simulink model "simu_pi"  (R2020b)
settings: Solver=VariableStepAuto  StartTime=0.0  StopTime=2  RelTol=1e-3
values from neighbouring files (symbols this model uses):
  K_p = 373.9-5    (= 368.9)    [ejemplo_1_pi.m]    (also in ejemplo_2_pid.m; zn.m = 9)
  T_i = K_p/2157.5    (= 0.170984936269)    [ejemplo_1_pi.m]    (also in ejemplo_2_pid.m; zn.m = 1.4)
settings Model: Creator=Acer  LastModifiedBy=Acer

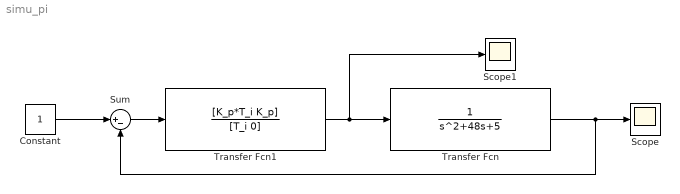
== system simu_pi ==
  Constant : Constant
  Scope : Scope
  Scope1 : Scope
  Sum : Sum  Inputs=|+-
  Transfer Fcn : TransferFcn  Denominator=[1 48 5]
  Transfer Fcn1 : TransferFcn  Numerator=[K_p*T_i K_p]  Denominator=[T_i 0]
  wires:
  Transfer Fcn1/1 -> Scope1/1, Transfer Fcn/1
  Transfer Fcn/1 -> Sum/2, Scope/1
  Sum/1 -> Transfer Fcn1/1
  Constant/1 -> Sum/1
